simulink model "Two_Stage_DTIADC_CTIADC"  (Simulink 10.0)
settings: Solver=ode45  StartTime=0.0  StopTime=100e-6  RelTol=1e-3  EnableMultiTasking=on
values from neighbouring files (symbols this model uses):
  a1 = 1/1    (= 1)    [Two_Stage_DTIADC_CTIADC_m.m]    (also in Two_Stage_IADC_m.m)
  a11 = 1/4    (= 0.25)    [Two_Stage_DTIADC_CTIADC_m.m]    (also in Two_Stage_IADC_m.m)
  a2 = 1/1    (= 1)    [Two_Stage_DTIADC_CTIADC_m.m]    (also in Two_Stage_IADC_m.m)
  adder_max = vref*1    (= 0.9)    [Two_Stage_DTIADC_CTIADC_m.m]    (also in Two_Stage_IADC_m.m)
  alfa = (opgain-1)/opgain    (= 0.999949881277)    [Two_Stage_DTIADC_CTIADC_m.m]    (also in Two_Stage_IADC_m.m)
  Amax = vref*1    (= 0.9)    [Two_Stage_DTIADC_CTIADC_m.m]    (also in Two_Stage_IADC_m.m)
  b11 = 4/1    (= 4)    [Two_Stage_DTIADC_CTIADC_m.m]    (also in Two_Stage_IADC_m.m)
  err_dac = 1.051/1000*0    (= 0)    [Two_Stage_DTIADC_CTIADC_m.m]    (also in Two_Stage_IADC_m.m)
  fs = OSR*fnyq    (= 12800000)    [Two_Stage_DTIADC_CTIADC_m.m]    (also in Two_Stage_IADC_m.m)
  fsig = 21.0e3    (= 21000)    [Two_Stage_DTIADC_CTIADC_m.m]    (also in Two_Stage_IADC_m.m)
  k1 = 1/1    (= 1)    [Two_Stage_DTIADC_CTIADC_m.m]    (also in Two_Stage_IADC_m.m)
  M = OSR-1    (= 127)    [Two_Stage_DTIADC_CTIADC_m.m]    (also in Two_Stage_IADC_m.m)
  mdac = [1 1 1 1  1 1 1 1]    [Two_Stage_DTIADC_CTIADC_m.m]    (also in Two_Stage_IADC_m.m)
  OSR = 64*2    (= 128)    [Two_Stage_DTIADC_CTIADC_m.m]    (also in Two_Stage_IADC_m.m)
  Tclk = Ts    (= 7.8125e-08)    [Two_Stage_DTIADC_CTIADC_m.m]
  Ts = 1/fs    (= 7.8125e-08)    [Two_Stage_DTIADC_CTIADC_m.m]    (also in Two_Stage_IADC_m.m)
  vin_amp = 10.^(vin_amp_db(index)/20)*vref    [Two_Stage_DTIADC_CTIADC_m.m]    (also in Two_Stage_IADC_m.m = 10.^(vin_amp_db/20)*vref)
  vref = 0.9    [Two_Stage_DTIADC_CTIADC_m.m]    (also in Two_Stage_IADC_m.m)
libraries: dspsigops x1
settings Model: LogicAnalyzerSignalOrdering=14ef830d-d328-4b55-81cf-95084106fef6,9e428476-7c6d-492d-b39c-22a694b9ca35,24752ac4-d810-4584-904c-a9f8ec941798,b366801f-0c4c-428c-8606-bd268a7e7b8e,00fdf89b-dfca-4d3f-a0e2-1f16acc85b46,ad35fcdc-dbf7-4935-a829-50dec5848964,65789b84-f8cb-42c7-ad3c-68f03d2abf26,69fd44d4-185a-4dc3-8e08-ae1d883c473b,17ea1185-1f64-4daf-8fc8-f56cb4bafa77,ff337881-3fa8-40ce-b00d-f2c13b67e4f3,cbaf1c38-494f-41b1-b01f-ddcafb799a33,afe8f8ad-ae3e-4305-afa0-25bef4a096ca,42f71387-198e-4e73-af2b-83bbd2b11719  Creator=chench  LastModifiedBy=benve
settings DataIOCC: LimitDataPoints=on
settings OptimizationCC: ExpressionDepthLimit=2147483647  InitFltsAndDblsToZero=on
settings DebuggingCC: SaveWithParameterizedLinksMsg=none  SignalResolutionControl=TryResolveAllWithWarning  SolverPrmCheckMsg=warning  MultiTaskDSMMsg=warning  MultiTaskCondExecSysMsg=none  FcnCallInpInsideContextMsg=warning  AllowSymbolicDim=off  StateNameClashWarn=warning
settings GRTTargetCC: TargetFcnLib=ansi_tfl_tmw.mat  GeneratePreprocessorConditionals=Disable all
settings ConfigComp: CovExternalEMLEnable=off

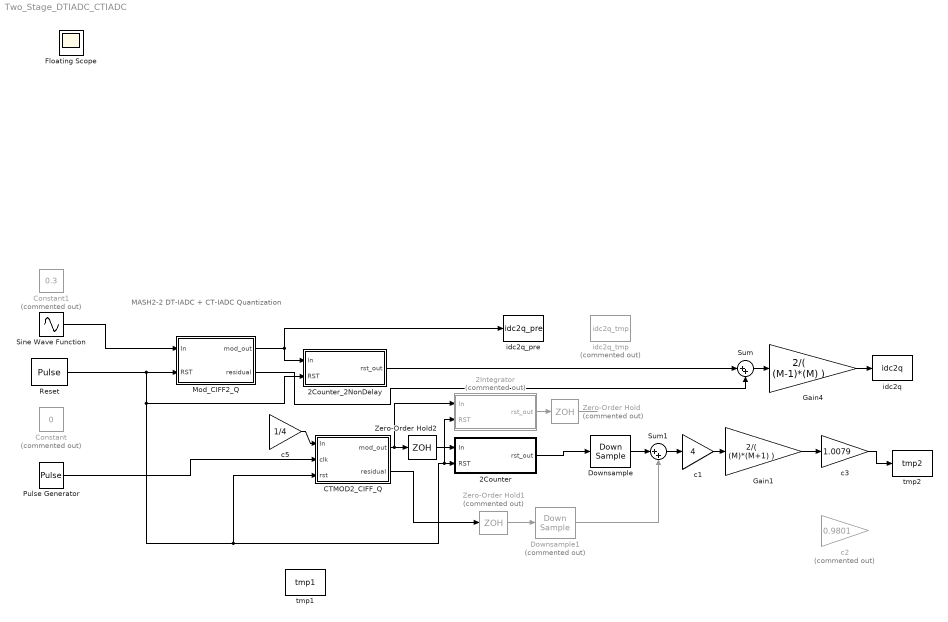
== system Two_Stage_DTIADC_CTIADC ==
  note: MASH2-2 DT-IADC + CT-IADC Quantization
  2Counter : Subsystem
  2Counter_2NonDelay : Subsystem
  2Integrator : Subsystem  Commented=on
  CTMOD2_CIFF_Q : Subsystem
  Constant : Constant  Commented=on  Value=0
  Constant1 : Constant  Commented=on  Value=0.3
  Downsample : DownSample  N=OSR  phase=OSR-1  RateOptions=Allow multirate processing
  Downsample1 : DownSample  Commented=on  N=OSR  phase=OSR-1  RateOptions=Allow multirate processing
  Gain1 : Gain  Gain=2/( (M)*(M+1) )
  Gain4 : Gain  Gain=2/( (M-1)*(M) )
  Mod_CIFF2_Q : Subsystem
  Pulse Generator : DiscretePulseGenerator  PulseType=Time based  Period=Ts  PulseWidth=50
  Reset : DiscretePulseGenerator  Period=OSR  SampleTime=Tclk
  Sine Wave Function : Sin  Amplitude=vin_amp  Frequency=fsig*2*pi  SampleTime=Tclk
  Sum : Sum  Inputs=|++
  Sum1 : Sum  Inputs=|++
  Zero-Order Hold : ZeroOrderHold  Commented=on  SampleTime=Ts
  Zero-Order Hold1 : ZeroOrderHold  Commented=on  SampleTime=Ts
  Zero-Order Hold2 : ZeroOrderHold  SampleTime=Ts
  c1 : Gain  Gain=4  SaturateOnIntegerOverflow=on  OutDataTypeStr=Inherit: Same as input  ParamDataTypeStr=Inherit: Same as input
  c2 : Gain  Commented=on  Gain=0.9801  SaturateOnIntegerOverflow=on  OutDataTypeStr=Inherit: Same as input  ParamDataTypeStr=Inherit: Same as input
  c3 : Gain  Gain=1.0079  SaturateOnIntegerOverflow=on  OutDataTypeStr=Inherit: Same as input  ParamDataTypeStr=Inherit: Same as input
  c5 : Gain  Gain=1/4  SaturateOnIntegerOverflow=on  OutDataTypeStr=Inherit: Same as input  ParamDataTypeStr=Inherit: Same as input
  idc2q : ToWorkspace  VariableName=idc2q  SampleTime=-1
  idc2q_pre : ToWorkspace  VariableName=idc2q_pre  SampleTime=-1
  idc2q_tmp : ToWorkspace  Commented=on  VariableName=idc2q_tmp  SampleTime=-1
  tmp1 : ToWorkspace  VariableName=tmp1  SampleTime=-1
  tmp2 : ToWorkspace  VariableName=tmp2  SampleTime=-1
  Floating Scope : Scope
  wires:
  Mod_CIFF2_Q/1(mod_out) -> 2Counter_2NonDelay/1(In), idc2q_pre/1
  Gain4/1 -> idc2q/1
  Sum/1 -> Gain4/1
  2Counter_2NonDelay/1(rst_out) -> Sum/1
  Sine Wave Function/1 -> Mod_CIFF2_Q/1(In)
  c5/1 -> CTMOD2_CIFF_Q/1(In)
  Zero-Order Hold2/1 -> 2Counter/1(In)
  Pulse Generator/1 -> CTMOD2_CIFF_Q/2(clk)
  Reset/1 -> 2Counter_2NonDelay/2(RST), 2Integrator/2(RST), 2Counter/2(RST), CTMOD2_CIFF_Q/3(rst), Mod_CIFF2_Q/2(RST)
  CTMOD2_CIFF_Q/1(mod_out) -> 2Integrator/1(In), Zero-Order Hold2/1
  Zero-Order Hold1/1 -> Downsample1/1
  CTMOD2_CIFF_Q/2(residual) -> Zero-Order Hold1/1
  c1/1 -> Gain1/1
  Downsample1/1 -> Sum1/2
  2Integrator/1(rst_out) -> Zero-Order Hold/1
  Sum1/1 -> c1/1
  Downsample/1 -> Sum1/1
  2Counter/1(rst_out) -> Downsample/1
  Zero-Order Hold/1 -> ?
  Gain1/1 -> c3/1
  c3/1 -> tmp2/1
  Mod_CIFF2_Q/2(residual) -> Sum/2

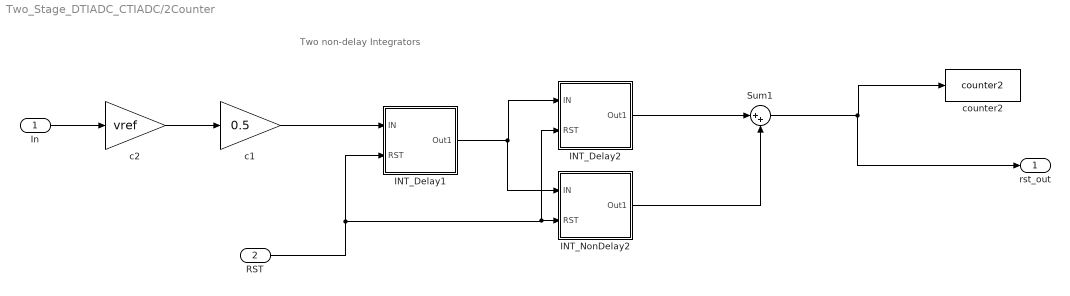
== system Two_Stage_DTIADC_CTIADC/2Counter ==
  note: Two non-delay Integrators
  In : Inport
  RST : Inport  Port=2
  INT_Delay1 : Subsystem
  INT_Delay2 : Subsystem
  INT_NonDelay2 : Subsystem
  Sum1 : Sum  Inputs=|++
  c1 : Gain  Gain=0.5  SaturateOnIntegerOverflow=on  OutDataTypeStr=Inherit: Same as input  ParamDataTypeStr=Inherit: Same as input
  c2 : Gain  Gain=vref  SaturateOnIntegerOverflow=on  OutDataTypeStr=Inherit: Same as input  ParamDataTypeStr=Inherit: Same as input
  counter2 : ToWorkspace  VariableName=counter2  SampleTime=-1
  rst_out : Outport  VectorParamsAs1DForOutWhenUnconnected=off
  wires:
  INT_Delay1/1(Out1) -> INT_NonDelay2/1(IN), INT_Delay2/1(IN)
  c1/1 -> INT_Delay1/1(IN)
  RST/1 -> INT_Delay1/2(RST), INT_NonDelay2/2(RST), INT_Delay2/2(RST)
  Sum1/1 -> rst_out/1, counter2/1
  In/1 -> c2/1
  INT_Delay2/1(Out1) -> Sum1/1
  INT_NonDelay2/1(Out1) -> Sum1/2
  c2/1 -> c1/1

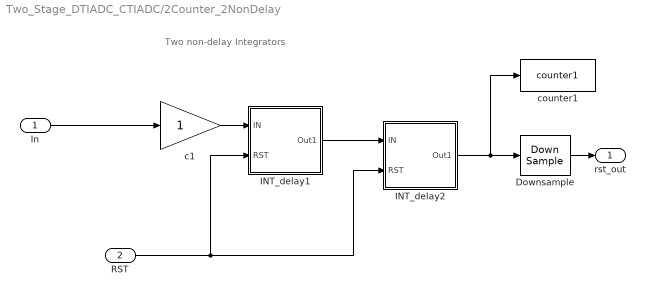
== system Two_Stage_DTIADC_CTIADC/2Counter_2NonDelay ==
  note: Two non-delay Integrators
  In : Inport
  RST : Inport  Port=2
  Downsample : DownSample  N=OSR  phase=OSR-1  RateOptions=Allow multirate processing
  INT_delay1 : Subsystem
  INT_delay2 : Subsystem
  c1 : Gain  SaturateOnIntegerOverflow=on  OutDataTypeStr=Inherit: Same as input  ParamDataTypeStr=Inherit: Same as input
  "counter1 " : ToWorkspace  VariableName=counter1  SampleTime=-1
  rst_out : Outport  VectorParamsAs1DForOutWhenUnconnected=off
  wires:
  INT_delay1/1(Out1) -> INT_delay2/1(IN)
  c1/1 -> INT_delay1/1(IN)
  INT_delay2/1(Out1) -> Downsample/1, "counter1 "/1
  RST/1 -> INT_delay1/2(RST), INT_delay2/2(RST)
  Downsample/1 -> rst_out/1
  In/1 -> c1/1

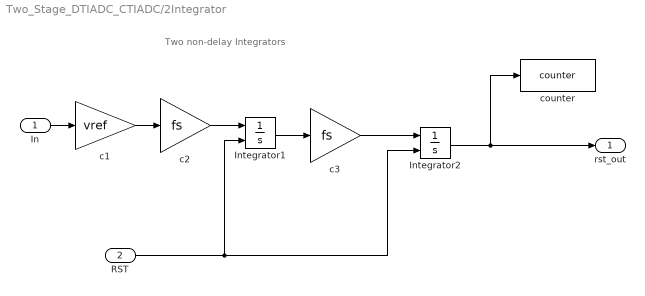
== system Two_Stage_DTIADC_CTIADC/2Integrator ==
  note: Two non-delay Integrators
  In : Inport
  RST : Inport  Port=2
  Integrator1 : Integrator  ExternalReset=rising
  Integrator2 : Integrator  ExternalReset=rising
  c1 : Gain  Gain=vref  SaturateOnIntegerOverflow=on  OutDataTypeStr=Inherit: Same as input  ParamDataTypeStr=Inherit: Same as input
  c2 : Gain  Gain=fs  SaturateOnIntegerOverflow=on  OutDataTypeStr=Inherit: Same as input  ParamDataTypeStr=Inherit: Same as input
  c3 : Gain  Gain=fs  SaturateOnIntegerOverflow=on  OutDataTypeStr=Inherit: Same as input  ParamDataTypeStr=Inherit: Same as input
  counter : ToWorkspace  VariableName=counter  SampleTime=-1
  rst_out : Outport  VectorParamsAs1DForOutWhenUnconnected=off
  wires:
  c1/1 -> c2/1
  RST/1 -> Integrator2/2, Integrator1/2
  Integrator2/1 -> rst_out/1, counter/1
  In/1 -> c1/1
  Integrator1/1 -> c3/1
  c2/1 -> Integrator1/1
  c3/1 -> Integrator2/1

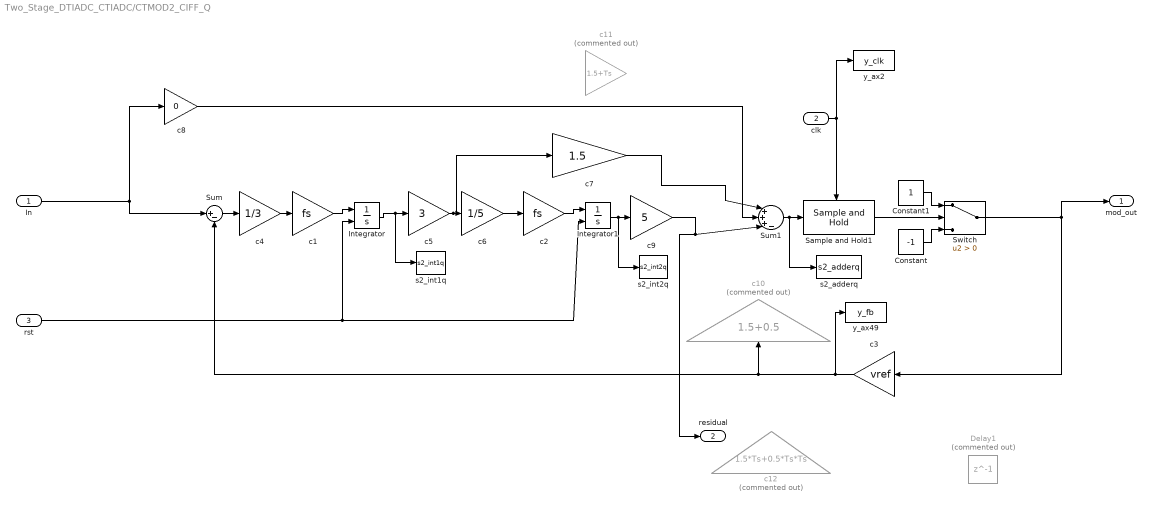
== system Two_Stage_DTIADC_CTIADC/CTMOD2_CIFF_Q ==
  In : Inport
  clk : Inport  Port=2
  rst : Inport  Port=3
  Constant : Constant  Value=-1
  Constant1 : Constant
  Delay1 : Delay  Commented=on  DelayLength=1  InitialCondition=0  SampleTime=Ts
  Integrator : Integrator  ExternalReset=rising
  Integrator1 : Integrator  ExternalReset=rising
  Sample and Hold1 : dspsigops/Sample and Hold  trig=Rising edge  initCond=0  latchinput=off
  Sum : Sum  Inputs=|+-
  Sum1 : Sum  Inputs=|+++-
  Switch : Switch  Criteria=u2 > Threshold
  c1 : Gain  Gain=fs  SaturateOnIntegerOverflow=on  OutDataTypeStr=Inherit: Same as input  ParamDataTypeStr=Inherit: Same as input
  c10 : Gain  Commented=on  Gain=1.5+0.5  SaturateOnIntegerOverflow=on  OutDataTypeStr=Inherit: Same as input  ParamDataTypeStr=Inherit: Same as input
  c11 : Gain  Commented=on  Gain=1.5+Ts  SaturateOnIntegerOverflow=on  OutDataTypeStr=Inherit: Same as input  ParamDataTypeStr=Inherit: Same as input
  c12 : Gain  Commented=on  Gain=1.5*Ts+0.5*Ts*Ts  SaturateOnIntegerOverflow=on  OutDataTypeStr=Inherit: Same as input  ParamDataTypeStr=Inherit: Same as input
  c2 : Gain  Gain=fs  SaturateOnIntegerOverflow=on  OutDataTypeStr=Inherit: Same as input  ParamDataTypeStr=Inherit: Same as input
  c3 : Gain  Gain=vref  SaturateOnIntegerOverflow=on  OutDataTypeStr=Inherit: Same as input  ParamDataTypeStr=Inherit: Same as input
  c4 : Gain  Gain=1/3  SaturateOnIntegerOverflow=on  OutDataTypeStr=Inherit: Same as input  ParamDataTypeStr=Inherit: Same as input
  c5 : Gain  Gain=3  SaturateOnIntegerOverflow=on  OutDataTypeStr=Inherit: Same as input  ParamDataTypeStr=Inherit: Same as input
  c6 : Gain  Gain=1/5  SaturateOnIntegerOverflow=on  OutDataTypeStr=Inherit: Same as input  ParamDataTypeStr=Inherit: Same as input
  c7 : Gain  Gain=1.5  SaturateOnIntegerOverflow=on  OutDataTypeStr=Inherit: Same as input  ParamDataTypeStr=Inherit: Same as input
  c8 : Gain  Gain=0  SaturateOnIntegerOverflow=on  OutDataTypeStr=Inherit: Same as input  ParamDataTypeStr=Inherit: Same as input
  c9 : Gain  Gain=5  SaturateOnIntegerOverflow=on  OutDataTypeStr=Inherit: Same as input  ParamDataTypeStr=Inherit: Same as input
  s2_adderq : ToWorkspace  VariableName=s2_adderq  SampleTime=-1
  s2_int1q : ToWorkspace  VariableName=s2_int1q  SampleTime=-1
  s2_int2q : ToWorkspace  VariableName=s2_int2q  SampleTime=-1
  y_ax2 : ToWorkspace  VariableName=y_clk  SaveFormat=Structure With Time  SampleTime=Ts/4
  y_ax49 : ToWorkspace  VariableName=y_fb  SaveFormat=Structure With Time  SampleTime=Ts/4
  mod_out : Outport  VectorParamsAs1DForOutWhenUnconnected=off
  residual : Outport  Port=2  VectorParamsAs1DForOutWhenUnconnected=off
  wires:
  In/1 -> Sum/1, c8/1
  c8/1 -> Sum1/2
  c7/1 -> Sum1/1
  Sum/1 -> c4/1
  Constant1/1 -> Switch/1
  Constant/1 -> Switch/3
  c5/1 -> c7/1, c6/1
  c9/1 -> residual/1, Sum1/3
  c4/1 -> c1/1
  c2/1 -> Integrator1/1
  c1/1 -> Integrator/1
  c6/1 -> c2/1
  Integrator1/1 -> s2_int2q/1, c9/1
  Integrator/1 -> s2_int1q/1, c5/1
  Sum1/1 -> s2_adderq/1, Sample and Hold1/1
  clk/1 -> Sample and Hold1/Trigger, y_ax2/1
  c3/1 -> Sum/2, c10/1, y_ax49/1
  Sample and Hold1/1 -> Switch/2
  Switch/1 -> c3/1, mod_out/1
  rst/1 -> Integrator1/2, Integrator/2

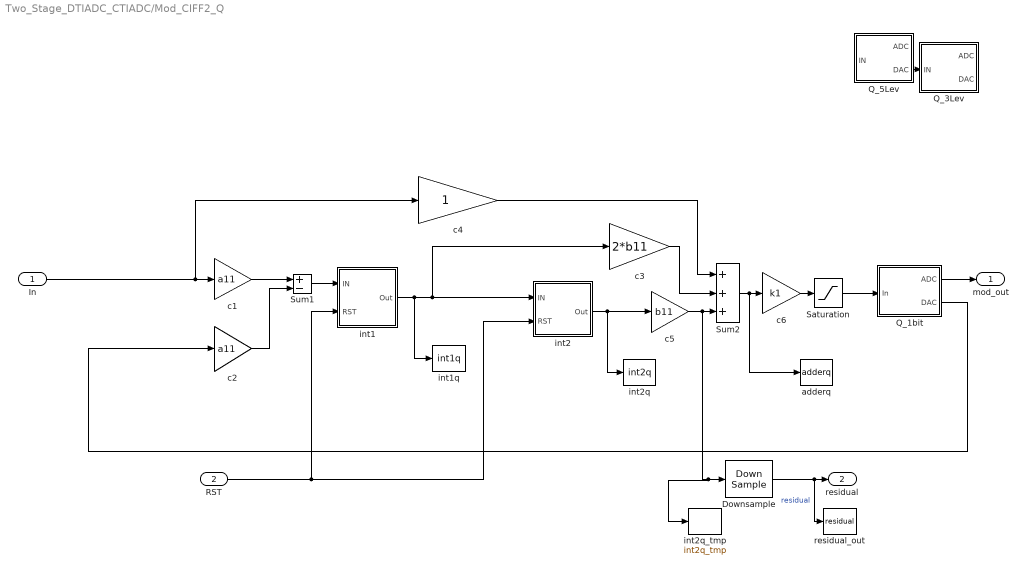
== system Two_Stage_DTIADC_CTIADC/Mod_CIFF2_Q ==
  In : Inport
  RST : Inport  Port=2
  Downsample : DownSample  N=OSR  phase=OSR-1  RateOptions=Allow multirate processing
  Q_1bit : Subsystem
  Q_3Lev : Subsystem
  Q_5Lev : Subsystem
  Saturation : Saturate  UpperLimit=adder_max*1  LowerLimit=-1*adder_max
  Sum1 : Sum  Inputs=+-  SaturateOnIntegerOverflow=on  InputSameDT=on  OutDataTypeStr=Inherit: Same as first input
  Sum2 : Sum  Inputs=+++  SaturateOnIntegerOverflow=on  InputSameDT=on  OutDataTypeStr=Inherit: Same as first input
  adderq : ToWorkspace  VariableName=adderq  SampleTime=-1
  c1 : Gain  Gain=a11  SaturateOnIntegerOverflow=on  OutDataTypeStr=Inherit: Same as input  ParamDataTypeStr=Inherit: Same as input
  c2 : Gain  Gain=a11  SaturateOnIntegerOverflow=on  OutDataTypeStr=Inherit: Same as input  ParamDataTypeStr=Inherit: Same as input
  c3 : Gain  Gain=2*b11  SaturateOnIntegerOverflow=on  OutDataTypeStr=Inherit: Same as input  ParamDataTypeStr=Inherit: Same as input
  c4 : Gain  SaturateOnIntegerOverflow=on  OutDataTypeStr=Inherit: Same as input  ParamDataTypeStr=Inherit: Same as input
  c5 : Gain  Gain=b11  SaturateOnIntegerOverflow=on  OutDataTypeStr=Inherit: Same as input  ParamDataTypeStr=Inherit: Same as input
  c6 : Gain  Gain=k1  SaturateOnIntegerOverflow=on  OutDataTypeStr=Inherit: Same as input  ParamDataTypeStr=Inherit: Same as input
  int1 : Subsystem
  int1q : ToWorkspace  VariableName=int1q  SampleTime=-1
  int2 : Subsystem
  int2q : ToWorkspace  VariableName=int2q  SampleTime=-1
  int2q_tmp : ToWorkspace  VariableName=int2q_tmp  SampleTime=-1
  residual_out : ToWorkspace  VariableName=residual  SampleTime=-1
  mod_out : Outport  VectorParamsAs1DForOutWhenUnconnected=off
  residual : Outport  Port=2  VectorParamsAs1DForOutWhenUnconnected=off
  wires:
  int1/1(Out) -> int1q/1, int2/1(IN), c3/1
  int2/1(Out) -> c5/1, int2q/1
  RST/1 -> int2/2(RST), int1/2(RST)
  c3/1 -> Sum2/2
  Saturation/1 -> Q_1bit/1(In)
  c5/1 -> int2q_tmp/1, Downsample/1, Sum2/3
  Q_1bit/1(ADC) -> mod_out/1
  c1/1 -> Sum1/1
  c2/1 -> Sum1/2
  In/1 -> c1/1, c4/1
  Sum1/1 -> int1/1(IN)
  c4/1 -> Sum2/1
  c6/1 -> Saturation/1
  Sum2/1 -> adderq/1, c6/1
  Q_1bit/2(DAC) -> c2/1
  Q_5Lev/2(DAC) -> Q_3Lev/1(IN)
  Downsample/1 -> residual_out/1, residual/1  "residual"

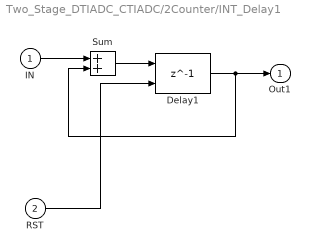
== system Two_Stage_DTIADC_CTIADC/2Counter/INT_Delay1 ==
  IN : Inport
  RST : Inport  Port=2
  Delay1 : Delay  DelayLength=1  InitialCondition=0  ExternalReset=Rising
      settings: InputPortMap=u0,r5
  Sum : Sum  SaturateOnIntegerOverflow=on  InputSameDT=on  OutDataTypeStr=Inherit: Same as first input
  Out1 : Outport  VectorParamsAs1DForOutWhenUnconnected=off
  wires:
  IN/1 -> Sum/1
  Sum/1 -> Delay1/1
  Delay1/1 -> Sum/2, Out1/1
  RST/1 -> Delay1/2

== system Two_Stage_DTIADC_CTIADC/2Counter/INT_Delay2 ==
  IN : Inport
  RST : Inport  Port=2
  Delay1 : Delay  DelayLength=1  InitialCondition=0  ExternalReset=Rising
      settings: InputPortMap=u0,r5
  Sum : Sum  SaturateOnIntegerOverflow=on  InputSameDT=on  OutDataTypeStr=Inherit: Same as first input
  Out1 : Outport  VectorParamsAs1DForOutWhenUnconnected=off
  wires:
  IN/1 -> Sum/1
  Sum/1 -> Delay1/1
  Delay1/1 -> Sum/2, Out1/1
  RST/1 -> Delay1/2

== system Two_Stage_DTIADC_CTIADC/2Counter/INT_NonDelay2 ==
  IN : Inport
  RST : Inport  Port=2
  Delay1 : Delay  DelayLength=1  InitialCondition=0  ExternalReset=Rising
      settings: InputPortMap=u0,r5
  Sum : Sum  SaturateOnIntegerOverflow=on  InputSameDT=on  OutDataTypeStr=Inherit: Same as first input
  Out1 : Outport  VectorParamsAs1DForOutWhenUnconnected=off
  wires:
  IN/1 -> Sum/1
  Sum/1 -> Delay1/1, Out1/1
  RST/1 -> Delay1/2
  Delay1/1 -> Sum/2

== system Two_Stage_DTIADC_CTIADC/2Counter_2NonDelay/INT_delay1 ==
  IN : Inport
  RST : Inport  Port=2
  Delay1 : Delay  DelayLength=1  InitialCondition=0  ExternalReset=Rising
      settings: InputPortMap=u0,r5
  Sum : Sum  SaturateOnIntegerOverflow=on  InputSameDT=on  OutDataTypeStr=Inherit: Same as first input
  Out1 : Outport  VectorParamsAs1DForOutWhenUnconnected=off
  wires:
  IN/1 -> Sum/1
  Sum/1 -> Delay1/1
  Delay1/1 -> Sum/2, Out1/1
  RST/1 -> Delay1/2

== system Two_Stage_DTIADC_CTIADC/2Counter_2NonDelay/INT_delay2 ==
  IN : Inport
  RST : Inport  Port=2
  Delay1 : Delay  DelayLength=1  InitialCondition=0  ExternalReset=Rising
      settings: InputPortMap=u0,r5
  Sum : Sum  SaturateOnIntegerOverflow=on  InputSameDT=on  OutDataTypeStr=Inherit: Same as first input
  Out1 : Outport  VectorParamsAs1DForOutWhenUnconnected=off
  wires:
  IN/1 -> Sum/1
  Sum/1 -> Delay1/1
  Delay1/1 -> Sum/2, Out1/1
  RST/1 -> Delay1/2

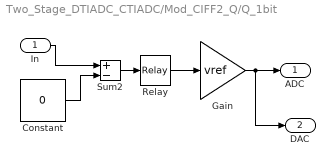
== system Two_Stage_DTIADC_CTIADC/Mod_CIFF2_Q/Q_1bit ==
  In : Inport
  Constant : Constant  Value=0
  Gain : Gain  Gain=vref
  Relay : Relay  OffOutputValue=-1  SampleTime=Tclk
  Sum2 : Sum  Inputs=+-  SaturateOnIntegerOverflow=on  InputSameDT=on  OutDataTypeStr=Inherit: Same as first input
  ADC : Outport  VectorParamsAs1DForOutWhenUnconnected=off
  DAC : Outport  Port=2  VectorParamsAs1DForOutWhenUnconnected=off
  wires:
  Sum2/1 -> Relay/1
  Constant/1 -> Sum2/2
  In/1 -> Sum2/1
  Relay/1 -> Gain/1
  Gain/1 -> ADC/1, DAC/1

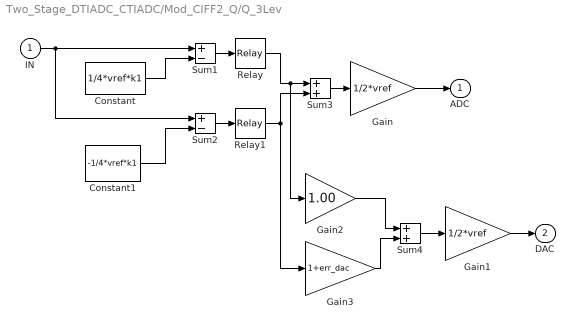
== system Two_Stage_DTIADC_CTIADC/Mod_CIFF2_Q/Q_3Lev ==
  IN : Inport
  Constant : Constant  Value=1/4*vref*k1
  Constant1 : Constant  Value=-1/4*vref*k1
  Gain : Gain  Gain=1/2*vref
  Gain1 : Gain  Gain=1/2*vref
  Gain2 : Gain  Gain=1.00
  Gain3 : Gain  Gain=1+err_dac
  Relay : Relay  OffOutputValue=-1  SampleTime=Tclk
  Relay1 : Relay  OffOutputValue=-1  SampleTime=Tclk
  Sum1 : Sum  Inputs=+-  SaturateOnIntegerOverflow=on  InputSameDT=on  OutDataTypeStr=Inherit: Same as first input
  Sum2 : Sum  Inputs=+-  SaturateOnIntegerOverflow=on  InputSameDT=on  OutDataTypeStr=Inherit: Same as first input
  Sum3 : Sum  SaturateOnIntegerOverflow=on  InputSameDT=on  OutDataTypeStr=Inherit: Same as first input
  Sum4 : Sum  SaturateOnIntegerOverflow=on  InputSameDT=on  OutDataTypeStr=Inherit: Same as first input
  ADC : Outport  VectorParamsAs1DForOutWhenUnconnected=off
  DAC : Outport  Port=2  VectorParamsAs1DForOutWhenUnconnected=off
  wires:
  Sum1/1 -> Relay/1
  Sum2/1 -> Relay1/1
  IN/1 -> Sum1/1, Sum2/1
  Constant/1 -> Sum1/2
  Constant1/1 -> Sum2/2
  Relay/1 -> Sum3/1, Gain2/1
  Relay1/1 -> Sum3/2, Gain3/1
  Sum3/1 -> Gain/1
  Gain/1 -> ADC/1
  Sum4/1 -> Gain1/1
  Gain2/1 -> Sum4/1
  Gain1/1 -> DAC/1
  Gain3/1 -> Sum4/2

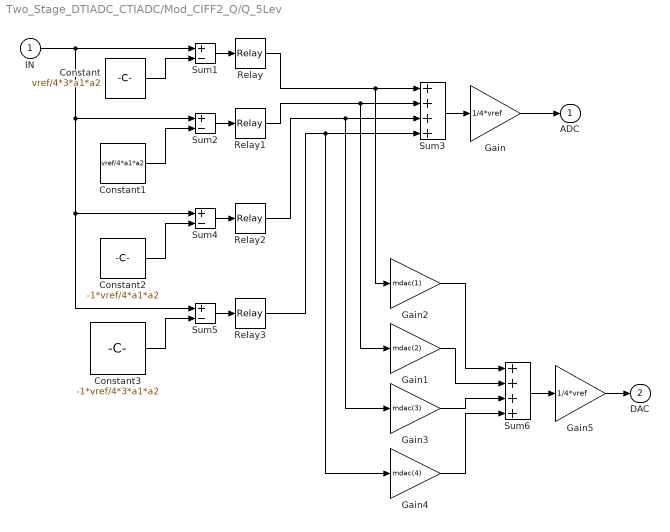
== system Two_Stage_DTIADC_CTIADC/Mod_CIFF2_Q/Q_5Lev ==
  IN : Inport
  Constant : Constant  Value=vref/4*3*a1*a2
  Constant1 : Constant  Value=vref/4*a1*a2
  Constant2 : Constant  Value=-1*vref/4*a1*a2
  Constant3 : Constant  Value=-1*vref/4*3*a1*a2
  Gain : Gain  Gain=1/4*vref
  Gain1 : Gain  Gain=mdac(2)
  Gain2 : Gain  Gain=mdac(1)
  Gain3 : Gain  Gain=mdac(3)
  Gain4 : Gain  Gain=mdac(4)
  Gain5 : Gain  Gain=1/4*vref
  Relay{,1..3} (4 alike) : Relay  OffOutputValue=-1  SampleTime=Tclk
  Sum{1..2,4..5} (4 alike) : Sum  Inputs=+-  SaturateOnIntegerOverflow=on  InputSameDT=on  OutDataTypeStr=Inherit: Same as first input
  Sum3 : Sum  Inputs=++++  SaturateOnIntegerOverflow=on  InputSameDT=on  OutDataTypeStr=Inherit: Same as first input
  Sum6 : Sum  Inputs=++++  SaturateOnIntegerOverflow=on  InputSameDT=on  OutDataTypeStr=Inherit: Same as first input
  ADC : Outport  VectorParamsAs1DForOutWhenUnconnected=off
  DAC : Outport  Port=2  VectorParamsAs1DForOutWhenUnconnected=off
  wires:
  Sum1/1 -> Relay/1
  Sum2/1 -> Relay1/1
  IN/1 -> Sum1/1, Sum2/1, Sum4/1, Sum5/1
  Constant/1 -> Sum1/2
  Constant1/1 -> Sum2/2
  Relay/1 -> Sum3/1, Gain2/1
  Relay1/1 -> Sum3/2, Gain1/1
  Sum3/1 -> Gain/1
  Gain/1 -> ADC/1
  Sum4/1 -> Relay2/1
  Constant2/1 -> Sum4/2
  Relay2/1 -> Sum3/3, Gain3/1
  Sum5/1 -> Relay3/1
  Constant3/1 -> Sum5/2
  Relay3/1 -> Sum3/4, Gain4/1
  Gain2/1 -> Sum6/1
  Gain1/1 -> Sum6/2
  Gain3/1 -> Sum6/3
  Gain4/1 -> Sum6/4
  Sum6/1 -> Gain5/1
  Gain5/1 -> DAC/1

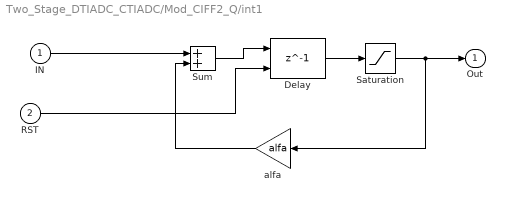
== system Two_Stage_DTIADC_CTIADC/Mod_CIFF2_Q/int1 ==
  IN : Inport
  RST : Inport  Port=2
  Delay : Delay  DelayLength=1  InitialCondition=0  ExternalReset=Rising
      settings: InputPortMap=u0,r5
  Saturation : Saturate  UpperLimit=Amax  LowerLimit=-1*Amax
  Sum : Sum  SaturateOnIntegerOverflow=on  InputSameDT=on  OutDataTypeStr=Inherit: Same as first input
  alfa : Gain  Gain=alfa  SaturateOnIntegerOverflow=on  OutDataTypeStr=Inherit: Same as input  ParamDataTypeStr=Inherit: Same as input
  Out : Outport  VectorParamsAs1DForOutWhenUnconnected=off
  wires:
  Delay/1 -> Saturation/1
  Saturation/1 -> Out/1, alfa/1
  Sum/1 -> Delay/1
  IN/1 -> Sum/1
  alfa/1 -> Sum/2
  RST/1 -> Delay/2

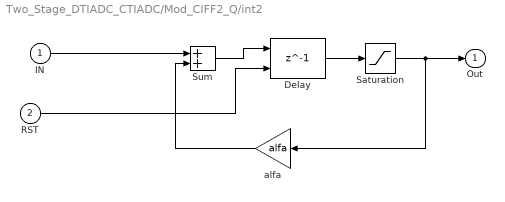
== system Two_Stage_DTIADC_CTIADC/Mod_CIFF2_Q/int2 ==
  IN : Inport
  RST : Inport  Port=2
  Delay : Delay  DelayLength=1  InitialCondition=0  ExternalReset=Rising
      settings: InputPortMap=u0,r5
  Saturation : Saturate  UpperLimit=Amax  LowerLimit=-1*Amax
  Sum : Sum  SaturateOnIntegerOverflow=on  InputSameDT=on  OutDataTypeStr=Inherit: Same as first input
  alfa : Gain  Gain=alfa  SaturateOnIntegerOverflow=on  OutDataTypeStr=Inherit: Same as input  ParamDataTypeStr=Inherit: Same as input
  Out : Outport  VectorParamsAs1DForOutWhenUnconnected=off
  wires:
  Delay/1 -> Saturation/1
  Saturation/1 -> Out/1, alfa/1
  Sum/1 -> Delay/1
  IN/1 -> Sum/1
  alfa/1 -> Sum/2
  RST/1 -> Delay/2
